simulink model "MPC"  (R2016a)
settings: Solver=VariableStepAuto  StartTime=0.0  StopTime=10.0  RelTol=1e-3
libraries: Meldas_library x2, mpclib x1
settings Model: Creator=Nam Bui Duy  LastModifiedBy=Nam Bui Duy

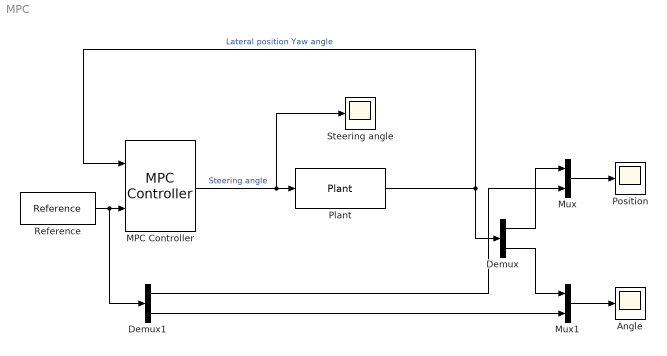
== system MPC ==
  Angle : Scope
  Demux : Demux  Outputs=2
  Demux1 : Demux  Outputs=2
  MPC Controller : mpclib/MPC Controller  SCDEnableBlockLinearizationSpecification=on  mpcobj=mpc1  is_multiple=0  enable_value=0  return_u0=off  ref_from_ws=off  ref_signal_name=[]  ref_preview=off  md_from_ws=off  md_signal_name=[]  md_preview=off  from_project=off  project_file=MPCtask.mat  md_inport=off  mv_inport=off  cost_outport=off  return_sequence=off  return_qpstatus=off  return_state=off  state_inport=off  lims_inport=off  ywt_inport=off  is_designfromscratch=0  uwt_inport=off  duwt_inport=off  rhoeps_inport=off  uref_inport=off  n_ts=0.1  n_mv=1  n_md=0  n_ud=0  n_mo=2  n_uo=0  BlockDataType=double  SampleTimeInherited=off  switch_inport=off
  Mux : Mux  Inputs=2
  Mux1 : Mux  Inputs=2
  Plant : Meldas_library/Plant  Vx=15
      mask Display: image('D:\MATLAB\Model-Predictive-Control-master\Car.jpg');
  Position : Scope
  Reference : Meldas_library/Reference  SystemSampleTime=-1
      mask Display: image('D:\MATLAB\Model-Predictive-Control-master\Reference.jpg');
  Steering angle : Scope
  wires:
  MPC Controller/1 -> Steering angle/1, Plant/1  "Steering angle"
  Plant/1 -> Demux/1, MPC Controller/1  "Lateral position Yaw angle"
  Reference/1 -> Demux1/1, MPC Controller/2
  Mux/1 -> Position/1
  Demux/1 -> Mux/1
  Demux1/1 -> Mux/2
  Mux1/1 -> Angle/1
  Demux/2 -> Mux1/1
  Demux1/2 -> Mux1/2
